simulink model "battery_with_sensors"  (R2022a)
settings: Solver=VariableStepAuto  StartTime=0.0  StopTime=10.0  RelTol=1e-3
undefined symbols (not defined in the file): Acid, Lead
libraries: spsBatteryLib x1, spsDiodeLib x1
settings Model: Creator=asher  LastModifiedBy=asher

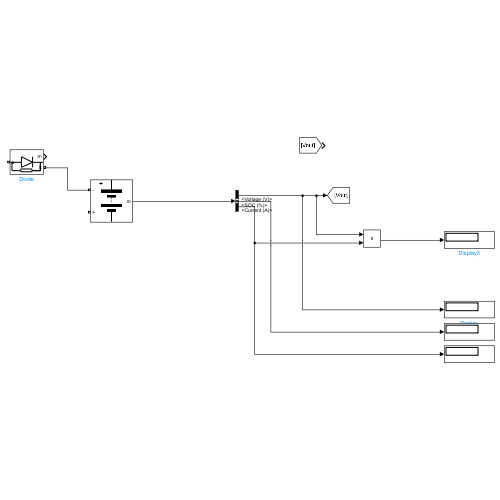
[thumbnail: Simulink's stored preview of the top-level diagram]
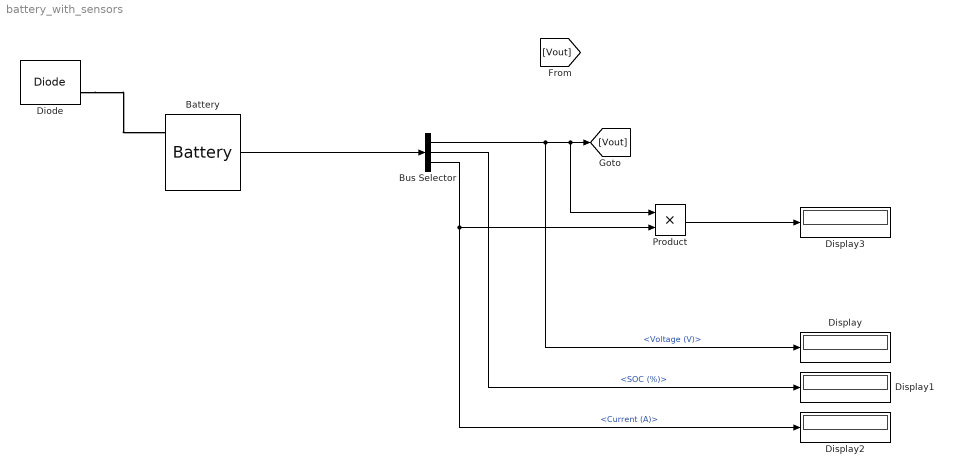
== system battery_with_sensors ==
  Battery : spsBatteryLib/Battery  BatType=Lead-Acid  ShowTempParam=off  ThermalPreset=no  ShowAgeParam=off  NomV=15  NomQ=100  SOC=100  Batt_Tr=1  PresetModel=on  MaxQ=104.1667  MinV=11.25  FullV=16.3322  Dis_rate=20  R=0.0015  Normal_OP=31.0278  expZone="[15.2714     0.333333]"  current=[6.5 13 32.5]  Units=Time  Tci=20  NomT=20  T2=-30  MaxQ2=4.8  FullV2=7.1  Normal_OP2=5.655  expZone2="[6.58           1]"  Rca=0.6  ti=2000  Dp=0  Neq0=0  Tsim=1e6  Ta1=25  Qeol=5.4*0.9  Reol=0.013333*1.2  Char_age=[2.3478, 3]  Dis_age=[2.3478, 10]  N1=1500  N2=10500  N3=1000  N4=1400  Ta2=45  N5=950
  Bus Selector : BusSelector  OutputSignals=Voltage (V),SOC (%),Current (A)
  Diode : spsDiodeLib/Diode  Ron=0.001  Lon=0  Vf=0.8  IC=0  UseSnubber=0  Rs=500  Cs=250e-9  Measurements=on
  Display{,1..3} (4 alike) : Display
  Product : Product
  wires:
  Battery/1 -> Bus Selector/1
  Bus Selector/1 -> Product/1, [Vout], Display/1  "<Voltage (V)>"
  Bus Selector/2 -> Display1/1  "<SOC (%)>"
  Bus Selector/3 -> Product/2, Display2/1  "<Current (A)>"
  Product/1 -> Display3/1
  connections:
  Diode/RConn1 -- Battery/LConn2
